simulink model "sampleModel1781"  (R2023a)
settings: Solver=VariableStepAuto  StartTime=0.0  StopTime=10.0  RelTol=1e-3
libraries: hdlsllib x2
settings Model: Creator=user1  LastModifiedBy=user1

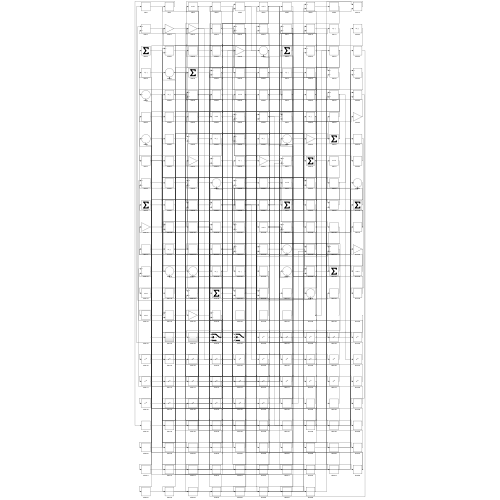
[thumbnail: Simulink's stored preview of the top-level diagram]
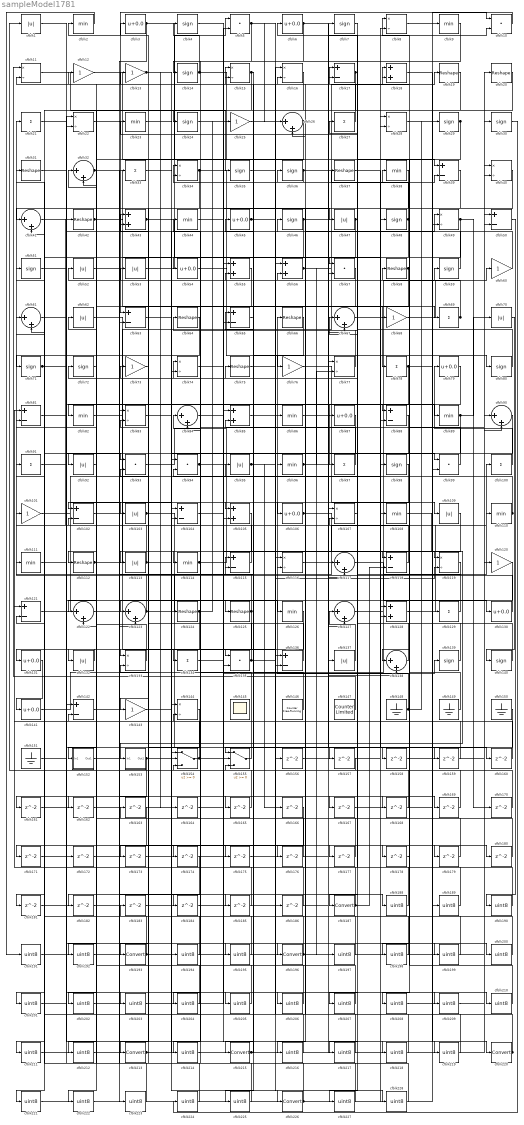
== system sampleModel1781 ==
  cfblk{1,47,52..53,62,70,92,95,103,109,113,132,137} (13 alike) : Abs  SaturateOnIntegerOverflow=off
  cfblk{5,10,57,93..94,99,135} (7 alike) : DotProduct  OutDataTypeStr=Inherit: Inherit via internal rule
  cfblk{21,27,33,69,78,91,97,100,129,134} (10 alike) : Sum  Inputs=+
  cfblk{12..13,25,60,68,73,76,101,120,143} (10 alike) : Gain
  cfblk{17,39,50,63,65,81,88,102,104,115,118,121,136,142} (14 alike) : Sum  Inputs=+-
  cfblk{18,43,55..56,85,105,128} (7 alike) : Sum
  cfblk{3,6,45,54,79,87,106,130..131,141} (10 alike) : Bias  Bias=0.0  SaturateOnIntegerOverflow=off
  cfblk{8,11,15..16,22,28,34,40,49,74,77,83,107,116,119,133,144} (17 alike) : Product  Inputs=*/  RndMeth=Zero  SaturateOnIntegerOverflow=on
  cfblk{2,9,23,38,44,82,86,89,96,108,110..111,114,126} (14 alike) : MinMax
  cfblk{19..20,31,37,42,58,64,66,75,112,124..125} (12 alike) : Reshape
  cfblk{26,32,41,61,67,84,90,117,122..123,127,138} (12 alike) : Sum  Inputs=|++
  cfblk{4,7,14,24,29..30,35..36,46,48,51,59,71..72,80,98,139..140} (18 alike) : Signum
  cfblk145 : Scope
      settings: Floating=on
  cfblk146 : hdlsllib/Sources/Counter Free-Running  NumBits=16  tsamp=-1
  cfblk147 : hdlsllib/Sources/Counter Limited  uplimit=7  tsamp=-1
  cfblk{148..151} (4 alike) : Ground
  cfblk152 : Subsystem
      settings: LibrarySourceBlock=|
      | hdlsllib/Ports &
      | Subsystems/Subsystem
  cfblk153 : Subsystem
      settings: LibrarySourceBlock=|
      | hdlsllib/Ports &
      | Subsystems/Subsystem
  cfblk154 : Switch  SaturateOnIntegerOverflow=off  InputSameDT=off
  cfblk155 : Switch  SaturateOnIntegerOverflow=off  InputSameDT=off
  cfblk{156..186} (31 alike) : Delay  SampleTime=1
  cfblk{187,193,196,213,215,220,226} (7 alike) : DataTypeConversion  SaturateOnIntegerOverflow=off  RndMeth=Floor
  cfblk{188..192,194..195,197..212,214,216..219,221..225,227..228} (35 alike) : DataTypeConversion  OutDataTypeStr=uint8  SaturateOnIntegerOverflow=off  RndMeth=Floor
  wires:
  cfblk53/1 -> cfblk5/1
  cfblk83/1 -> cfblk226/1
  cfblk76/1 -> cfblk109/1
  cfblk3/1 -> cfblk39/1, cfblk63/2
  cfblk56/1 -> cfblk18/1, cfblk197/1
  cfblk87/1 -> cfblk92/1
  cfblk113/1 -> cfblk42/1, cfblk179/1
  cfblk119/1 -> cfblk21/1
  cfblk10/1 -> cfblk63/1
  cfblk86/1 -> cfblk97/1
  cfblk127/1 -> cfblk59/1
  cfblk138/1 -> cfblk34/1
  cfblk15/1 -> cfblk162/1, cfblk225/1
  cfblk121/1 -> cfblk48/1
  cfblk93/1 -> cfblk85/2
  cfblk148/1 -> cfblk66/1, cfblk29/1
  cfblk147/1 -> cfblk11/1
  cfblk16/1 -> cfblk215/1
  cfblk135/1 -> cfblk2/1, cfblk119/2
  cfblk136/1 -> cfblk72/1
  cfblk150/1 -> cfblk155/1
  cfblk114/1 -> cfblk20/1, cfblk119/1
  cfblk97/1 -> cfblk52/1
  cfblk108/1 -> cfblk153/1(In1)
  cfblk27/1 -> cfblk11/2
  cfblk59/1 -> cfblk38/1
  cfblk13/1 -> cfblk65/2, cfblk164/1
  cfblk117/1 -> cfblk130/1
  cfblk95/1 -> cfblk166/1, cfblk167/1, cfblk168/1
  cfblk103/1 -> cfblk155/2, cfblk136/2
  cfblk34/1 -> cfblk80/1, cfblk113/1
  cfblk125/1 -> cfblk31/1, cfblk212/1
  cfblk112/1 -> cfblk19/1, cfblk178/1
  cfblk42/1 -> cfblk124/1, cfblk176/1
  cfblk25/1 -> cfblk136/1
  cfblk49/1 -> cfblk84/2, cfblk170/1, cfblk216/1
  cfblk62/1 -> cfblk135/1
  cfblk64/1 -> cfblk71/1
  cfblk36/1 -> cfblk39/2, cfblk34/2
  cfblk17/1 -> cfblk54/1, cfblk227/1
  cfblk58/1 -> cfblk122/1, cfblk208/1
  cfblk40/1 -> cfblk87/1
  cfblk79/1 -> cfblk82/1
  cfblk110/1 -> cfblk45/1, cfblk84/1
  cfblk65/1 -> cfblk15/1
  cfblk38/1 -> cfblk41/1
  cfblk106/1 -> cfblk118/1, cfblk117/2, cfblk189/1
  cfblk137/1 -> cfblk127/1
  cfblk71/1 -> cfblk88/1, cfblk88/2
  cfblk99/1 -> cfblk8/1
  cfblk51/1 -> cfblk46/1
  cfblk32/1 -> cfblk98/1, cfblk185/1
  cfblk28/1 -> cfblk220/1
  cfblk126/1 -> cfblk133/1
  cfblk100/1 -> cfblk79/1
  cfblk54/1 -> cfblk76/1
  cfblk98/1 -> cfblk132/1
  cfblk101/1 -> cfblk103/1
  cfblk124/1 -> cfblk134/1, cfblk25/1
  cfblk102/1 -> cfblk96/1
  cfblk141/1 -> cfblk100/1
  cfblk5/1 -> cfblk26/1, cfblk214/1, cfblk228/1
  cfblk82/1 -> cfblk154/1
  cfblk68/1 -> cfblk60/1
  cfblk57/1 -> cfblk102/1
  cfblk67/1 -> cfblk78/1
  cfblk4/1 -> cfblk47/1
  cfblk11/1 -> cfblk35/1
  cfblk122/1 -> cfblk33/1
  cfblk29/1 -> cfblk138/1, cfblk217/1
  cfblk69/1 -> cfblk18/2, cfblk43/2
  cfblk1/1 -> cfblk126/1
  cfblk43/1 -> cfblk108/1, cfblk99/1
  cfblk115/1 -> cfblk53/1
  cfblk120/1 -> cfblk213/1
  cfblk7/1 -> cfblk57/1
  cfblk66/1 -> cfblk105/1
  cfblk130/1 -> cfblk116/2
  cfblk14/1 -> cfblk86/1, cfblk4/1
  cfblk94/1 -> cfblk37/1, cfblk8/2
  cfblk96/1 -> cfblk77/2, cfblk159/1
  cfblk89/1 -> cfblk70/1, cfblk211/1
  cfblk44/1 -> cfblk68/1
  cfblk9/1 -> cfblk114/1
  cfblk85/1 -> cfblk89/1
  cfblk139/1 -> cfblk73/1
  cfblk61/1 -> cfblk196/1
  cfblk60/1 -> cfblk36/1
  cfblk12/1 -> cfblk105/2
  cfblk6/1 -> cfblk14/1, cfblk138/2, cfblk69/1, cfblk174/1
  cfblk144/1 -> cfblk193/1
  cfblk45/1 -> cfblk125/1, cfblk209/1
  cfblk80/1 -> cfblk23/1
  cfblk24/1 -> cfblk127/2
  cfblk129/1 -> cfblk6/1
  cfblk19/1 -> cfblk24/1
  cfblk73/1 -> cfblk123/1
  cfblk132/1 -> cfblk131/1
  cfblk123/1 -> cfblk110/1, cfblk12/1
  cfblk70/1 -> cfblk140/1
  cfblk8/1 -> cfblk10/1
  cfblk146/1 -> cfblk65/1
  cfblk154/1 -> cfblk139/1, cfblk43/1
  cfblk47/1 -> cfblk17/1, cfblk173/1
  cfblk140/1 -> cfblk64/1
  cfblk72/1 -> cfblk112/1
  cfblk128/1 -> cfblk40/2
  cfblk153/1(Out1) -> cfblk180/1, cfblk181/1
  cfblk118/1 -> cfblk41/2
  cfblk48/1 -> cfblk152/1(In1), cfblk27/1
  cfblk133/1 -> cfblk81/2
  cfblk131/1 -> cfblk141/1
  cfblk46/1 -> cfblk10/2, cfblk161/1
  cfblk77/1 -> cfblk56/2
  cfblk78/1 -> cfblk129/1, cfblk182/1
  cfblk149/1 -> cfblk17/2
  cfblk116/1 -> cfblk67/2
  cfblk31/1 -> cfblk93/1
  cfblk109/1 -> cfblk143/1
  cfblk39/1 -> cfblk106/1
  cfblk155/1 -> cfblk74/1
  cfblk143/1 -> cfblk49/1
  cfblk26/1 -> cfblk32/2, cfblk154/2
  cfblk107/1 -> cfblk187/1
  cfblk152/1(Out1) -> cfblk115/1
  cfblk75/1 -> cfblk156/1
  cfblk156/1 -> cfblk128/2
  cfblk41/1 -> cfblk157/1
  cfblk157/1 -> cfblk1/1
  cfblk63/1 -> cfblk158/1
  cfblk158/1 -> cfblk40/1
  cfblk159/1 -> cfblk102/2
  cfblk37/1 -> cfblk160/1
  cfblk160/1 -> cfblk81/1
  cfblk161/1 -> cfblk123/2
  cfblk162/1 -> cfblk85/1
  cfblk52/1 -> cfblk165/1
  cfblk165/1 -> cfblk93/2
  cfblk167/1 -> cfblk49/2
  cfblk168/1 -> cfblk26/2
  cfblk84/1 -> cfblk169/1
  cfblk169/1 -> cfblk155/3
  cfblk170/1 -> cfblk115/2
  cfblk20/1 -> cfblk171/1
  cfblk171/1 -> cfblk56/1
  cfblk21/1 -> cfblk172/1
  cfblk172/1 -> cfblk122/2
  cfblk173/1 -> cfblk57/2
  cfblk23/1 -> cfblk175/1
  cfblk175/1 -> cfblk77/1
  cfblk176/1 -> cfblk116/1
  cfblk134/1 -> cfblk177/1
  cfblk177/1 -> cfblk32/1
  cfblk179/1 -> cfblk154/3
  cfblk180/1 -> cfblk67/1
  cfblk181/1 -> cfblk74/2
  cfblk182/1 -> cfblk117/1
  cfblk105/1 -> cfblk184/1
  cfblk184/1 -> cfblk5/2
  cfblk185/1 -> cfblk121/1
  cfblk35/1 -> cfblk186/1
  cfblk186/1 -> cfblk133/2
  cfblk187/1 -> cfblk13/1, cfblk15/2, cfblk118/2
  cfblk164/1 -> cfblk188/1
  cfblk188/1 -> cfblk107/1
  cfblk189/1 -> cfblk107/2
  cfblk50/1 -> cfblk190/1
  cfblk190/1 -> cfblk101/1
  cfblk2/1 -> cfblk191/1
  cfblk191/1 -> cfblk50/1
  cfblk174/1 -> cfblk192/1
  cfblk192/1 -> cfblk50/2
  cfblk193/1 -> cfblk183/1, cfblk7/1
  cfblk33/1 -> cfblk194/1
  cfblk194/1 -> cfblk144/1
  cfblk151/1 -> cfblk195/1
  cfblk195/1 -> cfblk144/2
  cfblk196/1 -> cfblk44/1, cfblk51/1
  cfblk197/1 -> cfblk61/1
  cfblk178/1 -> cfblk198/1
  cfblk198/1 -> cfblk61/2
  cfblk22/1 -> cfblk199/1
  cfblk199/1 -> cfblk94/1
  cfblk18/1 -> cfblk200/1
  cfblk200/1 -> cfblk22/1
  cfblk88/1 -> cfblk201/1
  cfblk201/1 -> cfblk22/2
  cfblk163/1 -> cfblk202/1
  cfblk202/1 -> cfblk135/2
  cfblk91/1 -> cfblk203/1
  cfblk203/1 -> cfblk163/1
  cfblk55/1 -> cfblk204/1
  cfblk204/1 -> cfblk62/1
  cfblk81/1 -> cfblk205/1
  cfblk205/1 -> cfblk55/1
  cfblk183/1 -> cfblk206/1
  cfblk206/1 -> cfblk55/2
  cfblk90/1 -> cfblk207/1
  cfblk207/1 -> cfblk3/1
  cfblk208/1 -> cfblk90/1
  cfblk209/1 -> cfblk90/2
  cfblk104/1 -> cfblk210/1
  cfblk210/1 -> cfblk58/1
  cfblk211/1 -> cfblk104/1
  cfblk212/1 -> cfblk104/2
  cfblk213/1 -> cfblk99/2, cfblk137/1
  cfblk214/1 -> cfblk120/1
  cfblk215/1 -> cfblk95/1, cfblk30/1
  cfblk216/1 -> cfblk16/1
  cfblk217/1 -> cfblk16/2
  cfblk111/1 -> cfblk218/1
  cfblk218/1 -> cfblk128/1
  cfblk74/1 -> cfblk219/1
  cfblk219/1 -> cfblk111/1
  cfblk220/1 -> cfblk121/2, cfblk75/1
  cfblk166/1 -> cfblk221/1
  cfblk221/1 -> cfblk28/1
  cfblk92/1 -> cfblk222/1
  cfblk222/1 -> cfblk28/2
  cfblk142/1 -> cfblk223/1
  cfblk223/1 -> cfblk91/1
  cfblk30/1 -> cfblk224/1
  cfblk224/1 -> cfblk142/1
  cfblk225/1 -> cfblk142/2
  cfblk226/1 -> cfblk94/2, cfblk9/1
  cfblk227/1 -> cfblk83/1
  cfblk228/1 -> cfblk83/2

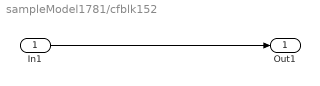
== system sampleModel1781/cfblk152 ==
  In1 : Inport
  Out1 : Outport
  wires:
  In1/1 -> Out1/1

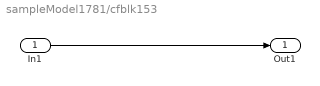
== system sampleModel1781/cfblk153 ==
  In1 : Inport
  Out1 : Outport
  wires:
  In1/1 -> Out1/1
